simulink model "Simulink lindo para imagenes"  (R2018a)
settings: Solver=VariableStepAuto  StartTime=0.0  StopTime=10.0  RelTol=1e-3
undefined symbols (not defined in the file): F, Kint, pint
settings Model: Creator=54249  LastModifiedBy=54249

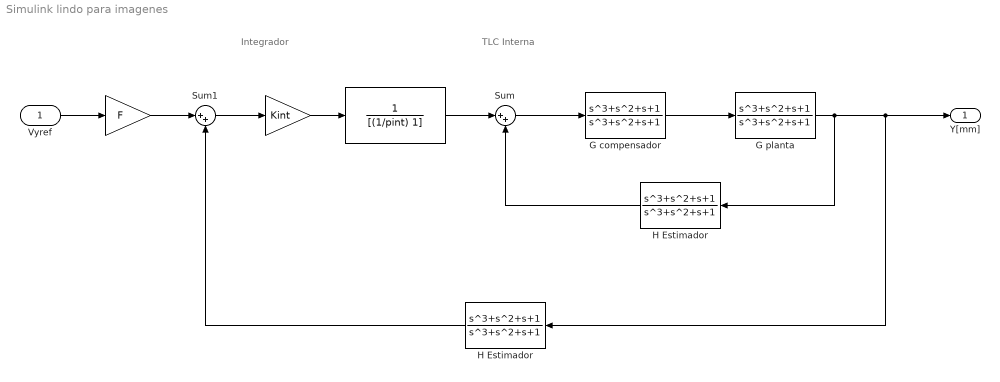
== system Simulink lindo para imagenes ==
  note: Integrador
  note: TLC Interna
  Vyref : Inport
  " " : Gain  Gain=Kint
  " " : Gain  Gain=F
  " " : TransferFcn  Denominator=[(1/pint) 1]
  "G compensador " : TransferFcn  Numerator=[1 1 1 1]  Denominator=[1 1 1 1]
  "G planta " : TransferFcn  Numerator=[1 1 1 1]  Denominator=[1 1 1 1]
  H Estimador : TransferFcn  Numerator=[1 1 1 1]  Denominator=[1 1 1 1]
  "H Estimador " : TransferFcn  Numerator=[1 1 1 1]  Denominator=[1 1 1 1]
  Sum : Sum  Inputs=|++
  Sum1 : Sum  Inputs=|++
  Y[mm] : Outport
  wires:
  Sum1/1 -> " "/1
  " "/1 -> " "/1
  " "/1 -> Sum/1
  " "/1 -> Sum1/1
  Sum/1 -> "G compensador "/1
  "G compensador "/1 -> "G planta "/1
  "G planta "/1 -> "H Estimador "/1, H Estimador/1, Y[mm]/1
  "H Estimador "/1 -> Sum/2
  H Estimador/1 -> Sum1/2
  Vyref/1 -> " "/1
